simulink model "Ex4"  (R2024b)
settings: Solver=VariableStepAuto  StartTime=0.0  StopTime=30  RelTol=1e-3
values from neighbouring files (symbols this model uses):
  A = [0 1 0 0 0 0;-(K1+K2+K3)/M1 -(C1+C2+C3)/M1 K2/M1 C2/M1 K3/M1 C3/M1;     0 0 0 1 0 0; K2/M2 C2/M2 -(K2+K4+K5)/M2 -(C2+C4+C5)/M2 K4/M2 C4/M2;     0 0 0 0 0 1;K5/M3 C3/M3 K4/M3 C4/M3 -(K3+K4)/M3 -(C3+C4)/M3]    [Tp1.m]
  Ao = A-L*C_x2    [Tp1.m]
  B = [0; 0; 0 ; 1/M2; 0; 0 ]    [Tp1.m]
  Bo = [B L]    [Tp1.m]
  C = [eye(6)]    [Tp1.m]
  C_x2 = [0 0 1 0 0 0]    [Tp1.m]
  Co = eye(6)    [Tp1.m]
  D = [0;0;0;0;0;0]    [Tp1.m]
  Do = [0 0 0 0 0 0; 0 0 0 0 0 0]'    [Tp1.m]
  Kr = lqr(A,B,Q,R)    [Tp1.m]
  x0 = [x10;0;x20;0;x30;0]    [Tp1.m]
settings Model: Creator=Pedro Mendes
settings RTWCC: GPUComputeCapability=3.5

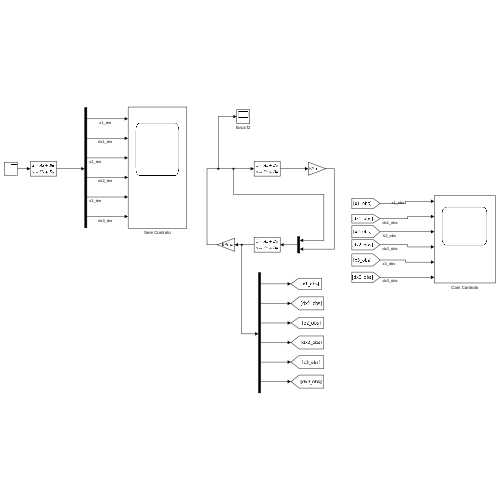
[thumbnail: Simulink's stored preview of the top-level diagram]
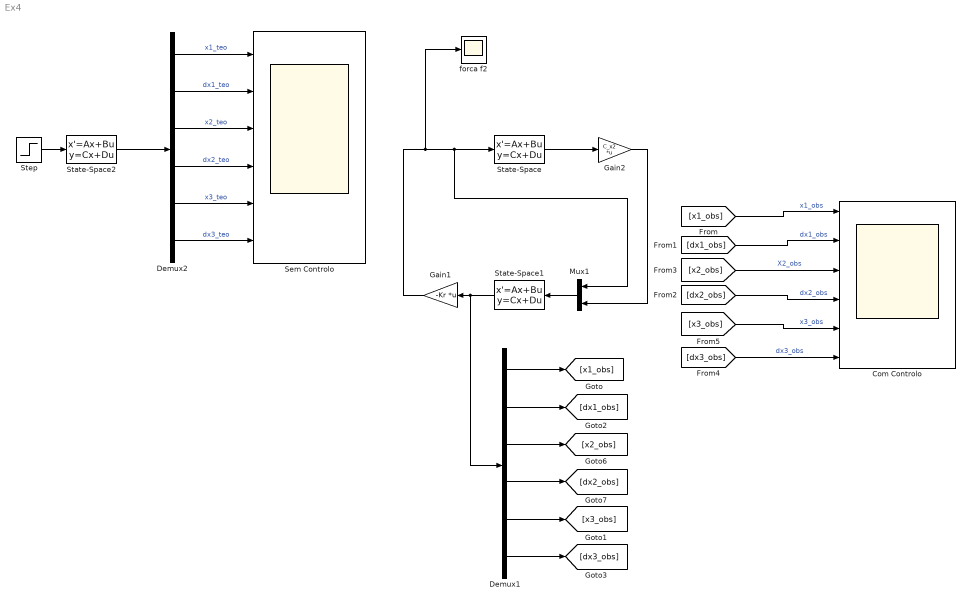
== system Ex4 ==
  Com Controlo : Scope  NumInputPorts=6
  Demux1 : Demux  Outputs=6
  Demux2 : Demux  Outputs=6
  Gain1 : Gain  Gain=-Kr  Multiplication=Matrix(K*u) (u vector)
  Gain2 : Gain  Gain=C_x2  Multiplication=Matrix(K*u)
  Mux1 : Mux  Inputs=2
  Sem Controlo : Scope  NumInputPorts=6
  State-Space : StateSpace  A=A  B=B  C=C  D=D  InitialCondition=x0
  State-Space1 : StateSpace  A=Ao  B=Bo  C=Co  D=Do  InitialCondition=0  ParameterTunability=Optimized
  State-Space2 : StateSpace  A=A  B=B  C=C  D=D  InitialCondition=x0
  Step : Step  SampleTime=0
  forca f2 : Scope
  wires:
  State-Space1/1 -> Demux1/1, Gain1/1
  Mux1/1 -> State-Space1/1
  Gain1/1 -> forca f2/1, Mux1/1, State-Space/1
  Demux1/1 -> [x1_obs]
  [x1_obs] -> Com Controlo/1  "x1_obs"
  Demux1/2 -> [dx1_obs]
  State-Space/1 -> Gain2/1
  Gain2/1 -> Mux1/2
  Step/1 -> State-Space2/1
  Demux1/6 -> [dx3_obs]
  Demux1/5 -> [x3_obs]
  Demux1/4 -> [dx2_obs]
  Demux1/3 -> [x2_obs]
  State-Space2/1 -> Demux2/1
  Demux2/1 -> Sem Controlo/1  "x1_teo"
  Demux2/2 -> Sem Controlo/2  "dx1_teo"
  Demux2/3 -> Sem Controlo/3  "x2_teo"
  Demux2/4 -> Sem Controlo/4  "dx2_teo"
  Demux2/5 -> Sem Controlo/5  "x3_teo"
  Demux2/6 -> Sem Controlo/6  "dx3_teo"
  [dx1_obs] -> Com Controlo/2  "dx1_obs"
  [x2_obs] -> Com Controlo/3  "X2_obs"
  [dx2_obs] -> Com Controlo/4  "dx2_obs"
  [x3_obs] -> Com Controlo/5  "x3_obs"
  [dx3_obs] -> Com Controlo/6  "dx3_obs"
